simulink model "cv_model_F50"  (R2023a)
settings: Solver=ode23t  StartTime=0  StopTime=6000  FixedStep=0.0005  MaxStep=.01  RelTol=1e-4
model workspace (MAT data in the model file):
  test = 0
values from neighbouring files (symbols this model uses):
  A_cheb_09_1 = [-9.45889157397 1 0 0 0 0 0 0 0 -116.684730988 0 1 ... (81 elements, 9x9)]    [input_reflex_filters.mat]
  B_cheb_09_1 = [1 0 0 0 0 0 0 0 0]    [input_reflex_filters.mat]
  C_cheb_09_1 = [0 0 0 0 0 0 0 0 151338.279895]    [input_reflex_filters.mat]
libraries: SignalEditorBlockLib x4, simulink_extras x4
(part 3 of 4)

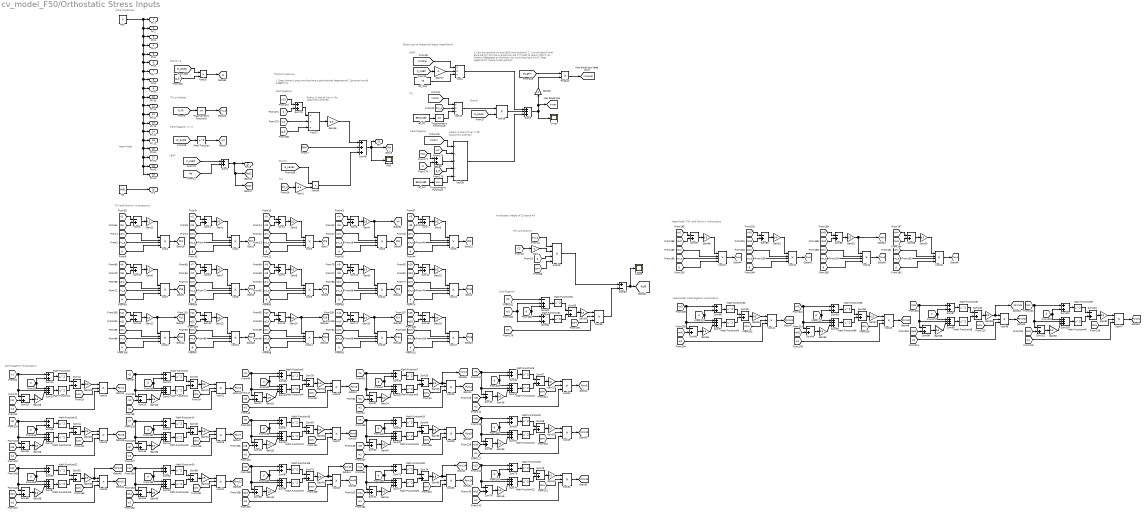
== system cv_model_F50/Orthostatic Stress Inputs ==
  note: Head Model
  note: Centrifugation
  note: Tilt (and Gravity)
  note: Gravity
  note: Tilt
  note: LBNP
  note: Centrifugation
  note: Radius is that of liver (ri for splanchnic arteries).
  note: Gravity
  note: Tilt
  note: Centrifugation: Hydrostatics
  note: 1. Can we combine tilt and LBNP contributions?
      | 2. I've included G level because this formula is empirical, but it stands to reason that if you tilted to 85degrees on the Moon you would lose less fluid
      | 3. Does negative tilt induce hypervolemia?
  note: Hydrostatic Height of CS above AA
  note: Blood Lost to Interstitial Space (Head Down)
  note: Tilt: sin(alpha)
  note: Tilt (and Gravity): Hydrostatics
  note: Initial Conditions
  note: LBNP
  note: Thoracic Pressure
  note: 1. Does thoracic pressure drop have a gravitational dependence? Zamanian would suggest so.
  note: Centrifugation: w^2
  note: Gravity: g
  note: Centrifugation
  note: Radius is that of liver (ri for splanchnic arteries).
  note: Head Model: Tillt (and Gravity) Hydrostatics
  note: Head Model: Centrifugation Hydrostatics
  Gain : Gain  Gain=-1
  Gain1 : Gain  Gain=-3.5  SaturateOnIntegerOverflow=on  OutDataTypeStr=Inherit: Same as input  ParamDataTypeStr=Inherit: Same as input
  Gain{2,5..12,15..16,18..21,23,25..39,41,43..47,49..61} (50 alike) : Gain  Gain=0.5  SaturateOnIntegerOverflow=on  OutDataTypeStr=Inherit: Same as input  ParamDataTypeStr=Inherit: Same as input
  Gain{3..4,13..14,22,24,40,42} (8 alike) : Gain  Gain=1/3  SaturateOnIntegerOverflow=on  OutDataTypeStr=Inherit: Same as input  ParamDataTypeStr=Inherit: Same as input
  Gain17 : Gain  Gain=-1  SaturateOnIntegerOverflow=on  OutDataTypeStr=Inherit: Same as input  ParamDataTypeStr=Inherit: Same as input
  Gain48 : Gain  Gain=-3.5  SaturateOnIntegerOverflow=on  OutDataTypeStr=Inherit: Same as input  ParamDataTypeStr=Inherit: Same as input
  Gain62 : Gain  Gain=-1
  Math Function{,1..40} (41 alike) : Math  Operator=square
  Ph0 : Constant  Value=0
  Product : Product
  Pth1 : Scope
  R0 : Constant  Value=.0001
  Scope : Scope
  Sum{1,4..13,15..19,21,23,25,27,29,31,33,35,37,39,41,43,46,48,50,52,54,56,58,60,62,64,66,68,70,72,74,76,78,83,85..88,90,92,94,96,98,100,102,104} (58 alike) : Sum  Inputs=-+  InputSameDT=on  SaturateOnIntegerOverflow=on  OutDataTypeStr=Inherit: Same as first input
  Sum{2,14,22,26,30,34,38,42,47,51,55,59,63,67,71,75,79..80,84,89,93,97,101} (23 alike) : Sum  InputSameDT=on  SaturateOnIntegerOverflow=on  OutDataTypeStr=Inherit: Same as first input
  Sum{3,20,24,28,32,36,40,44..45,49,53,57,61,65,69,73,77,91,95,99,103} (21 alike) : Sum  Inputs=+++  InputSameDT=on  SaturateOnIntegerOverflow=on  OutDataTypeStr=Inherit: Same as first input
  Sum81 : Sum  Inputs=+-  InputSameDT=on  SaturateOnIntegerOverflow=on  OutDataTypeStr=Inherit: Same as first input
  Sum82 : Sum  Inputs=-++  InputSameDT=on  SaturateOnIntegerOverflow=on  OutDataTypeStr=Inherit: Same as first input
  Trigonometric Function1 : Trigonometry
  Trigonometric Function16 : Trigonometry
  Trigonometric Function2 : Trigonometry
  Vmax : Scope
  kool{1..3,5..14,16..17,19,40..43} (20 alike) : Product  Inputs=****  InputSameDT=on  SaturateOnIntegerOverflow=on  OutDataTypeStr=Inherit: Same as first input
  kool15 : Product  Inputs=**/  InputSameDT=on  SaturateOnIntegerOverflow=on  OutDataTypeStr=Inherit: Same as first input
  kool18 : Product  Inputs=**  InputSameDT=on  SaturateOnIntegerOverflow=on  OutDataTypeStr=Inherit: Same as first input
  kool{20..34,39,44..47} (20 alike) : Product  Inputs=3  InputSameDT=on  SaturateOnIntegerOverflow=on  OutDataTypeStr=Inherit: Same as first input
  kool35 : Product  Inputs=**  InputSameDT=on  SaturateOnIntegerOverflow=on  OutDataTypeStr=Inherit: Same as first input
  kool36 : Product  Inputs=**  InputSameDT=on  SaturateOnIntegerOverflow=on  OutDataTypeStr=Inherit: Same as first input
  kool37 : Product  Inputs=**/  InputSameDT=on  SaturateOnIntegerOverflow=on  OutDataTypeStr=Inherit: Same as first input
  kool38 : Product  Inputs=***//  InputSameDT=on  SaturateOnIntegerOverflow=on  OutDataTypeStr=Inherit: Same as first input
  kool4 : Product  Inputs=**/  InputSameDT=on  SaturateOnIntegerOverflow=on  OutDataTypeStr=Inherit: Same as first input
  ref_lbnp : Constant  Value=70
  ref_src : Constant  Value=85*pi/180
  ref_tilt : Constant  Value=85*pi/180
  Ph.1 : Outport
  Ph.2 : Outport  Port=2
  Ph.3 : Outport  Port=3
  Ph.4 : Outport  Port=4
  Ph.5 : Outport  Port=5
  Ph.6 : Outport  Port=6
  Ph.7 : Outport  Port=7
  Ph.8 : Outport  Port=8
  Ph.9 : Outport  Port=9
  Ph.10 : Outport  Port=10
  Ph.11 : Outport  Port=11
  Ph.12 : Outport  Port=12
  Ph.13 : Outport  Port=13
  Ph.14 : Outport  Port=14
  Ph.15 : Outport  Port=15
  Ph.H1 : Outport  Port=16
  Ph.H2 : Outport  Port=17
  Ph.H3 : Outport  Port=18
  Ph.H4 : Outport  Port=19
  R.0 : Outport  Port=20
  Pth : Outport  Port=21
  Pe.LB : Outport  Port=22
  tag scope: Pe12=global, Pe13=global, Ph10=global, Ph11=global, Ph12=global, Ph13=global, Ph14=global, Ph15=global, Ph1=global, Ph2=global, Ph3=global, Ph4=global, Ph5=global, Ph6=global, Ph7=global, Ph8=global, Ph9=global, PhH1=global, PhH2=global, PhH3=global, PhH4=global, Poff=global, Psrc10=global, Psrc11=global, Psrc12=global, Psrc13=global, Psrc14=global, Psrc15=global, Psrc1=global, Psrc2=global, Psrc3=global, Psrc4=global, Psrc5=global, Psrc6=global, Psrc7=global, Psrc8=global, Psrc9=global, PsrcH1=global, PsrcH2=global, PsrcH3=global, PsrcH4=global, Pth=global, Vmax=global, Vmaxub=global, g=global, h11=global, h13=global, h14=global, h4=global, hH3=global, hsrc11=global, hsrc13=global, hsrc14=global, hsrc4=global, hsrcH3=global, sin_a=global, w2=global
  wires:
  Ph0/1 -> Ph.8/1, Ph.H4/1, Ph.H3/1, Ph.H2/1, Ph.H1/1, Ph.15/1, Ph.14/1, Ph.13/1, Ph.12/1, Ph.11/1, Ph.10/1, Ph.9/1, Ph.7/1, Ph.6/1, Ph.5/1, Ph.4/1, Ph.3/1, Ph.2/1, Ph.1/1
  R0/1 -> R.0/1
  ref_tilt/1 -> Trigonometric Function16/1
  [Vmtilt] -> kool15/1
  Trigonometric Function16/1 -> kool15/3
  [conv] -> kool1/2
  [sin_a] -> kool1/3
  [ri1] -> Sum5/1
  [sin_a] -> kool19/1
  [g] -> kool19/3
  Trigonometric Function2/1 -> [sin_a]
  Gain11/1 -> kool1/1
  Gain/1 -> kool19/2
  [conv] -> kool19/4
  [g] -> kool1/4
  [P_TA] -> Trigonometric Function2/1
  kool1/1 -> [Ph1]
  Sum5/1 -> Gain11/1
  [ro1] -> Sum5/2
  [g] -> kool2/4
  [ri2] -> Sum1/1
  kool2/1 -> [Ph2]
  [conv] -> kool2/2
  [sin_a] -> kool2/3
  Gain2/1 -> kool2/1
  [ro2] -> Sum1/2
  Sum1/1 -> Gain2/1
  Sum4/1 -> Gain3/1
  kool3/1 -> [Ph3]
  [ri3] -> Sum4/1
  [conv] -> kool3/2
  [sin_a] -> kool3/3
  Gain3/1 -> kool3/1
  [ro3] -> Sum4/2
  [g] -> kool3/4
  [g] -> kool5/4
  kool5/1 -> [Ph4]
  Gain4/1 -> [h4], kool5/1
  [ri4] -> Sum6/1
  [sin_a] -> kool5/3
  [ro4] -> Sum6/2
  Sum6/1 -> Gain4/1
  [conv] -> kool5/2
  [sin_a] -> kool6/3
  [ro5] -> Sum7/2
  [ri5] -> Sum7/1
  Gain5/1 -> kool6/1
  [conv] -> kool6/2
  kool6/1 -> [Ph5]
  Sum7/1 -> Gain5/1
  [g] -> kool6/4
  [conv] -> kool10/2
  [ri9] -> Sum11/1
  Gain9/1 -> kool10/1
  kool10/1 -> [Ph9]
  [ri10] -> Sum12/1
  [ro10] -> Sum12/2
  kool11/1 -> [Ph10]
  [g] -> kool10/4
  Sum10/1 -> Gain6/1
  [conv] -> kool11/2
  [ri6] -> Sum10/1
  [g] -> kool9/4
  Gain10/1 -> kool11/1
  [ro8] -> Sum9/2
  Sum11/1 -> Gain9/1
  [conv] -> kool9/2
  [sin_a] -> kool7/3
  kool9/1 -> [Ph8]
  [g] -> kool7/4
  Sum12/1 -> Gain10/1
  Gain8/1 -> kool9/1
  [ri8] -> Sum9/1
  [sin_a] -> kool9/3
  Sum9/1 -> Gain8/1
  kool7/1 -> [Ph6]
  [conv] -> kool7/2
  [sin_a] -> kool10/3
  [ro9] -> Sum11/2
  [g] -> kool11/4
  Gain6/1 -> kool7/1
  [ro6] -> Sum10/2
  Sum8/1 -> Gain7/1
  [sin_a] -> kool11/3
  kool8/1 -> [Ph7]
  [ri7] -> Sum8/1
  [conv] -> kool8/2
  [sin_a] -> kool8/3
  Gain7/1 -> kool8/1
  [ro7] -> Sum8/2
  [g] -> kool8/4
  [conv] -> kool16/2
  [ri14] -> Sum17/1
  Gain15/1 -> [h14], kool16/1
  kool16/1 -> [Ph14]
  [ri15] -> Sum18/1
  [ro15] -> Sum18/2
  kool17/1 -> [Ph15]
  [g] -> kool16/4
  Sum16/1 -> Gain12/1
  [conv] -> kool17/2
  [ri11] -> Sum16/1
  [g] -> kool14/4
  Gain16/1 -> kool17/1
  [ro13] -> Sum15/2
  Sum17/1 -> Gain15/1
  [conv] -> kool14/2
  [sin_a] -> kool12/3
  kool14/1 -> [Ph13]
  [g] -> kool12/4
  Sum18/1 -> Gain16/1
  Gain14/1 -> [h13], kool14/1
  [ri13] -> Sum15/1
  [sin_a] -> kool14/3
  Sum15/1 -> Gain14/1
  kool12/1 -> [Ph11]
  [conv] -> kool12/2
  [sin_a] -> kool16/3
  [ro14] -> Sum17/2
  [g] -> kool17/4
  Gain12/1 -> kool12/1, [h11]
  [ro11] -> Sum16/2
  Sum13/1 -> Gain13/1
  [sin_a] -> kool17/3
  kool13/1 -> [Ph12]
  [ri12] -> Sum13/1
  [conv] -> kool13/2
  [sin_a] -> kool13/3
  Gain13/1 -> kool13/1
  [ro12] -> Sum13/2
  [g] -> kool13/4
  [sin_a] -> Gain1/1
  [sin_a] -> kool15/2
  Sum2/1 -> [Pe13], [Pe12], Pe.LB/1
  [P_LNBP] -> Sum2/1
  [Pe] -> Sum2/2
  [CS] -> Gain/1
  Gain17/1 -> kool4/2
  [Vmlbnp] -> kool4/1
  ref_lbnp/1 -> kool4/3
  Sum3/1 -> Gain62/1, [Vmax], Vmax/1
  kool4/1 -> Sum3/1
  [P_LNBP] -> Gain17/1
  kool15/1 -> kool18/1
  [G_LEVEL] -> kool18/2
  kool18/1 -> Sum3/2
  Math Function/1 -> [w2]
  [W_RADS] -> Math Function/1
  kool20/1 -> [Psrc1]
  [ro1] -> Sum19/2
  Sum19/1 -> Gain18/1
  [ri1] -> Sum14/1, Sum19/1, Sum20/2
  [d] -> Sum20/1, Sum14/2
  Gain18/1 -> Sum20/3
  Sum14/1 -> Math Function1/1
  Sum20/1 -> Math Function2/1
  Math Function2/1 -> Sum21/2
  Math Function1/1 -> Sum21/1
  Sum21/1 -> Gain19/1
  Gain19/1 -> kool20/1
  [conv] -> kool20/2
  [w2] -> kool20/3
  [conv] -> kool21/2
  Sum23/1 -> Gain20/1
  [w2] -> kool21/3
  Sum25/1 -> Gain21/1
  Sum22/1 -> Math Function3/1
  Gain20/1 -> Sum24/3
  Math Function3/1 -> Sum25/1
  Sum24/1 -> Math Function4/1
  kool21/1 -> [Psrc2]
  [ri2] -> Sum22/1, Sum23/1, Sum24/2
  Gain21/1 -> kool21/1
  Math Function4/1 -> Sum25/2
  [ro2] -> Sum23/2
  [d] -> Sum24/1, Sum22/2
  Gain23/1 -> kool22/1
  [ri3] -> Sum26/1, Sum27/1, Sum28/2
  Gain22/1 -> Sum28/3
  Sum28/1 -> Math Function6/1
  Sum26/1 -> Math Function5/1
  Math Function5/1 -> Sum29/1
  Sum29/1 -> Gain23/1
  [d] -> Sum28/1, Sum26/2
  [conv] -> kool22/2
  Sum27/1 -> Gain22/1
  [w2] -> kool22/3
  kool22/1 -> [Psrc3]
  Math Function6/1 -> Sum29/2
  [ro3] -> Sum27/2
  Gain25/1 -> [hsrc4], kool23/1
  [ri4] -> Sum30/1, Sum31/1, Sum32/2
  Gain24/1 -> Sum32/3
  Sum32/1 -> Math Function8/1
  Sum30/1 -> Math Function7/1
  Math Function7/1 -> Sum33/1
  Sum33/1 -> Gain25/1
  [d] -> Sum32/1, Sum30/2
  [conv] -> kool23/2
  Sum31/1 -> Gain24/1
  [w2] -> kool23/3
  kool23/1 -> [Psrc4]
  Math Function8/1 -> Sum33/2
  [ro4] -> Sum31/2
  Gain27/1 -> kool24/1
  [ri5] -> Sum34/1, Sum35/1, Sum36/2
  Gain26/1 -> Sum36/3
  Sum36/1 -> Math Function10/1
  Sum34/1 -> Math Function9/1
  Math Function9/1 -> Sum37/1
  Sum37/1 -> Gain27/1
  [d] -> Sum36/1, Sum34/2
  [conv] -> kool24/2
  Sum35/1 -> Gain26/1
  [w2] -> kool24/3
  kool24/1 -> [Psrc5]
  Math Function10/1 -> Sum37/2
  [ro5] -> Sum35/2
  [ro6] -> Sum39/2
  [conv] -> kool25/2
  Gain28/1 -> Sum40/3
  Sum39/1 -> Gain28/1
  [w2] -> kool25/3
  Sum41/1 -> Gain29/1
  Sum38/1 -> Math Function11/1
  Math Function11/1 -> Sum41/1
  Sum47/1 -> Math Function16/1
  [ri8] -> Sum47/1, Sum48/1, Sum49/2
  Sum49/1 -> Math Function17/1
  Math Function16/1 -> Sum50/1
  Sum50/1 -> Gain33/1
  Gain32/1 -> Sum49/3
  Gain33/1 -> kool27/1
  Math Function13/1 -> Sum41/2
  [conv] -> kool27/2
  [d] -> Sum49/1, Sum47/2
  Math Function17/1 -> Sum50/2
  [ro8] -> Sum48/2
  Sum48/1 -> Gain32/1
  kool29/1 -> [Psrc10]
  Math Function12/1 -> Sum58/2
  [ro10] -> Sum56/2
  [w2] -> kool29/3
  Math Function20/1 -> Sum58/1
  Sum57/1 -> Math Function12/1
  kool27/1 -> [Psrc8]
  Gain36/1 -> Sum57/3
  Sum56/1 -> Gain36/1
  [d] -> Sum57/1, Sum55/2
  kool25/1 -> [Psrc6]
  [d] -> Sum53/1, Sum51/2
  [conv] -> kool29/2
  kool28/1 -> [Psrc9]
  [conv] -> kool28/2
  Sum52/1 -> Gain34/1
  Gain34/1 -> Sum53/3
  Sum54/1 -> Gain35/1
  Sum51/1 -> Math Function18/1
  Gain35/1 -> kool28/1
  Gain37/1 -> kool29/1
  [w2] -> kool28/3
  [ri7] -> Sum42/1, Sum43/1, Sum44/2
  Math Function19/1 -> Sum54/2
  Gain30/1 -> Sum44/3
  Sum55/1 -> Math Function20/1
  Sum44/1 -> Math Function15/1
  Sum42/1 -> Math Function14/1
  Sum53/1 -> Math Function19/1
  Math Function14/1 -> Sum46/1
  Sum46/1 -> Gain31/1
  Math Function18/1 -> Sum54/1
  [w2] -> kool26/3
  kool26/1 -> [Psrc7]
  Sum43/1 -> Gain30/1
  [ri6] -> Sum38/1, Sum39/1, Sum40/2
  Gain31/1 -> kool26/1
  [d] -> Sum44/1, Sum42/2
  Math Function15/1 -> Sum46/2
  Sum58/1 -> Gain37/1
  [ri10] -> Sum55/1, Sum56/1, Sum57/2
  Sum40/1 -> Math Function13/1
  [ro7] -> Sum43/2
  Gain29/1 -> kool25/1
  [ro9] -> Sum52/2
  [d] -> Sum40/1, Sum38/2
  [ri9] -> Sum51/1, Sum52/1, Sum53/2
  [conv] -> kool26/2
  [w2] -> kool27/3
  [ro11] -> Sum60/2
  [conv] -> kool30/2
  Gain38/1 -> Sum61/3
  Sum60/1 -> Gain38/1
  [w2] -> kool30/3
  Sum62/1 -> Gain39/1
  Sum59/1 -> Math Function21/1
  Math Function21/1 -> Sum62/1
  Sum67/1 -> Math Function26/1
  [ri13] -> Sum67/1, Sum68/1, Sum69/2
  Sum69/1 -> Math Function27/1
  Math Function26/1 -> Sum70/1
  Sum70/1 -> Gain43/1
  Gain42/1 -> Sum69/3
  Gain43/1 -> [hsrc13], kool32/1
  Math Function23/1 -> Sum62/2
  [conv] -> kool32/2
  [d] -> Sum69/1, Sum67/2
  Math Function27/1 -> Sum70/2
  [ro13] -> Sum68/2
  Sum68/1 -> Gain42/1
  kool34/1 -> [Psrc15]
  Math Function22/1 -> Sum78/2
  [ro15] -> Sum76/2
  [w2] -> kool34/3
  Math Function30/1 -> Sum78/1
  Sum77/1 -> Math Function22/1
  kool32/1 -> [Psrc13]
  Gain46/1 -> Sum77/3
  Sum76/1 -> Gain46/1
  [d] -> Sum77/1, Sum75/2
  kool30/1 -> [Psrc11]
  [d] -> Sum73/1, Sum71/2
  [conv] -> kool34/2
  kool33/1 -> [Psrc14]
  [conv] -> kool33/2
  Sum72/1 -> Gain44/1
  Gain44/1 -> Sum73/3
  Sum74/1 -> Gain45/1
  Sum71/1 -> Math Function28/1
  Gain45/1 -> [hsrc14], kool33/1
  Gain47/1 -> kool34/1
  [w2] -> kool33/3
  [ri12] -> Sum63/1, Sum64/1, Sum65/2
  Math Function29/1 -> Sum74/2
  Gain40/1 -> Sum65/3
  Sum75/1 -> Math Function30/1
  Sum65/1 -> Math Function25/1
  Sum63/1 -> Math Function24/1
  Sum73/1 -> Math Function29/1
  Math Function24/1 -> Sum66/1
  Sum66/1 -> Gain41/1
  Math Function28/1 -> Sum74/1
  [w2] -> kool31/3
  kool31/1 -> [Psrc12]
  Sum64/1 -> Gain40/1
  [ri11] -> Sum59/1, Sum60/1, Sum61/2
  Gain41/1 -> kool31/1
  [d] -> Sum65/1, Sum63/2
  Math Function25/1 -> Sum66/2
  Sum78/1 -> Gain47/1
  [ri15] -> Sum75/1, Sum76/1, Sum77/2
  Sum61/1 -> Math Function23/1
  [ro12] -> Sum64/2
  Gain39/1 -> [hsrc11], kool30/1
  [ro14] -> Sum72/2
  [d] -> Sum61/1, Sum59/2
  [ri14] -> Sum71/1, Sum72/1, Sum73/2
  [conv] -> kool31/2
  [w2] -> kool32/3
  [G_LEVEL] -> kool35/1
  [g_E] -> kool35/2
  kool35/1 -> [g]
  Gain1/1 -> kool36/2
  [G_LEVEL] -> kool36/1
  [Pth0] -> Sum45/2
  kool36/1 -> Sum45/3
  Sum45/1 -> Pth1/1, [Pth], Pth/1
  [g_E] -> kool37/3
  [w2] -> kool37/2
  Sum79/1 -> kool37/1
  [ri10] -> Sum79/1
  [d] -> Sum79/2
  Gain48/1 -> Sum45/1
  kool37/1 -> Gain48/1
  [w2] -> kool38/2
  [Vmsrc] -> kool38/1
  ref_src/1 -> Trigonometric Function1/1
  Sum80/1 -> kool38/3
  [g_E] -> kool38/4
  Trigonometric Function1/1 -> kool38/5
  [ri10] -> Sum80/1
  [d] -> Sum80/2
  kool38/1 -> Sum3/3
  Sum81/1 -> Scope/1, [Poff]
  kool19/1 -> Sum81/1
  Sum84/1 -> Math Function31/1
  [ro1] -> Sum82/2, Sum84/2
  Sum85/1 -> Gain50/1
  Sum82/1 -> Math Function32/1
  Math Function31/1 -> Sum85/2
  Gain50/1 -> kool39/1
  [d] -> Sum84/1, Sum82/3
  [conv] -> kool39/2
  kool39/1 -> Sum81/2
  [w2] -> kool39/3
  Math Function32/1 -> Sum85/1
  [CS] -> Sum82/1
  kool40/1 -> [PhH1]
  kool43/1 -> [PhH4]
  [conv] -> kool42/2
  [riH2] -> Sum83/1
  Gain53/1 -> kool43/1
  [sin_a] -> kool40/3
  [riH3] -> Sum86/1
  Gain51/1 -> kool41/1
  [roH1] -> Sum87/2
  kool41/1 -> [PhH2]
  [roH3] -> Sum86/2
  Sum83/1 -> Gain51/1
  [riH1] -> Sum87/1
  [roH4] -> Sum88/2
  [conv] -> kool41/2
  [conv] -> kool40/2
  [sin_a] -> kool43/3
  [g] -> kool43/4
  [sin_a] -> kool41/3
  Gain52/1 -> [hH3], kool42/1
  [g] -> kool42/4
  [conv] -> kool43/2
  [sin_a] -> kool42/3
  Gain49/1 -> kool40/1
  [riH4] -> Sum88/1
  kool42/1 -> [PhH3]
  [roH2] -> Sum83/2
  Sum86/1 -> Gain52/1
  [g] -> kool41/4
  [g] -> kool40/4
  Sum87/1 -> Gain49/1
  Sum88/1 -> Gain53/1
  [conv] -> kool47/2
  Sum99/1 -> Math Function38/1
  Sum91/1 -> Math Function34/1
  [w2] -> kool47/3
  Gain60/1 -> Sum103/3
  [w2] -> kool44/3
  Math Function38/1 -> Sum100/2
  [d] -> Sum103/1, Sum101/2
  [conv] -> kool45/2
  Sum92/1 -> Gain55/1
  [w2] -> kool46/3
  Sum98/1 -> Gain58/1
  kool47/1 -> [PsrcH4]
  Sum93/1 -> Math Function35/1
  Math Function39/1 -> Sum104/1
  Sum101/1 -> Math Function39/1
  Gain61/1 -> kool47/1
  Sum95/1 -> Math Function36/1
  Gain56/1 -> Sum95/3
  Sum100/1 -> Gain59/1
  [riH4] -> Sum101/1, Sum102/1, Sum103/2
  [conv] -> kool46/2
  Sum97/1 -> Math Function37/1
  Gain58/1 -> Sum99/3
  [roH4] -> Sum102/2
  Sum102/1 -> Gain60/1
  kool46/1 -> [PsrcH3]
  Sum103/1 -> Math Function40/1
  [d] -> Sum95/1, Sum93/2
  Math Function37/1 -> Sum100/1
  [roH3] -> Sum98/2
  [riH3] -> Sum97/1, Sum98/1, Sum99/2
  Math Function36/1 -> Sum96/2
  Gain57/1 -> kool45/1
  [conv] -> kool44/2
  Gain59/1 -> [hsrcH3], kool46/1
  kool44/1 -> [PsrcH1]
  [roH2] -> Sum94/2
  Sum89/1 -> Math Function33/1
  Gain54/1 -> Sum91/3
  Math Function34/1 -> Sum92/2
  Math Function35/1 -> Sum96/1
  kool45/1 -> [PsrcH2]
  Math Function40/1 -> Sum104/2
  [d] -> Sum91/1, Sum89/2
  [d] -> Sum99/1, Sum97/2
  [riH1] -> Sum89/1, Sum90/1, Sum91/2
  Sum96/1 -> Gain57/1
  Gain55/1 -> kool44/1
  [w2] -> kool45/3
  Sum90/1 -> Gain54/1
  [riH2] -> Sum93/1, Sum94/1, Sum95/2
  Math Function33/1 -> Sum92/1
  Sum104/1 -> Gain61/1
  [roH1] -> Sum90/2
  Sum94/1 -> Gain56/1
  Product/1 -> [Vmaxub]
  Gain62/1 -> Product/2
  [ub_gain] -> Product/1

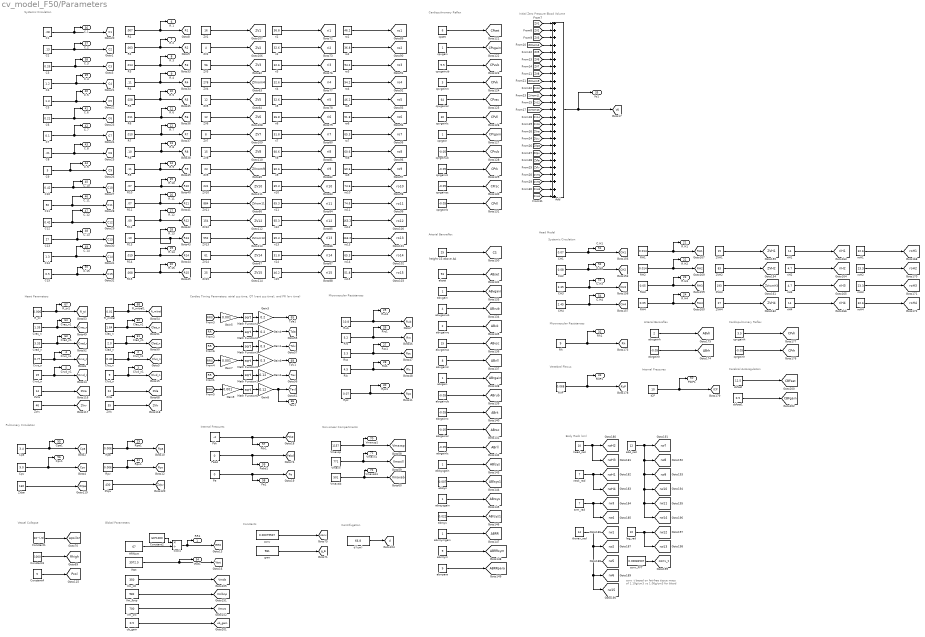
== system cv_model_F50/Parameters ==
  note: Arterial Baroreflex
  note: Systemic Circulation
  note: Microvascular Resistances
  note: Initial Zero Pressure Blood Volume
  note: Cardiopulmonary Reflex
  note: Centrifugation
  note: Constants
  note: Vessel Collapse
  note: Non-Linear Compartments
  note: Heart Parameters
  note: Cardiac Timing Parameters: atrial sys time, QT (vent sys time), and PR (a-v time)
  note: Internal Pressures
  note: Pulmonary Circulation
  note: Microvascular Resistances
  note: Global Parameters
  note: Systemic Circulation
  note: Arterial Baroreflex
  note: Head Model
  note: Cardiopulmonary Reflex
  note: Vertebral Plexus
  note: Internal Pressures
  note: Body Radii (cm)
  note: conv_t based on fat-free tissue mass of 1.10g/cm3 vs 1.06g/cm3 for blood
  note: Cerebral Autoregulation
  Add : Sum  Inputs=+++++++++++++++++++++++++
  C1 : Constant  Value=.28
  C10 : Constant  Value=0.42
  C11 : Constant  Value=50
  C12 : Constant  Value=0.42
  C13 : Constant  Value=27
  C14 : Constant  Value=1.3
  C15 : Constant  Value=0.5
  C2 : Constant  Value=.13
  C3 : Constant  Value=0.26
  C4 : Constant  Value=1.2
  C5 : Constant  Value=1.3
  C6 : Constant  Value=0.21
  C7 : Constant  Value=0.1
  C8 : Constant  Value=.21
  C9 : Constant  Value=5
  CH1 : Constant  Value=0.07
  CH2 : Constant  Value=0.08
  CH3 : Constant  Value=3.35
  CH4 : Constant  Value=2.45
  Clad_n : Constant  Value=2.0
  Clas_n : Constant  Value=1.64
  Clvd_n : Constant  Value=9
  Clvs_n : Constant  Value=0.40
  Constant1 : Constant  Value=10^(-5)
  Constant2 : Constant  Value=60*1000
  Constant3 : Constant  Value=1000
  Constant4 : Constant  Value=5
  Cpa : Constant  Value=3.4
  Cpv : Constant  Value=9.0
  Crad_n : Constant  Value=3.33
  Cras_n : Constant  Value=1.35
  Crvd_n : Constant  Value=19
  Crvs_n : Constant  Value=0.77
  Gain1 : Gain  Gain=0.3
  Gain2 : Gain  Gain=0.12
  Gain3 : Gain  Gain=0.2
  Gain4 : Gain  Gain=0.2
  Gain5 : Gain  Gain=0.001
  Gain6 : Gain  Gain=0.3
  Gain7 : Gain  Gain=0.001
  Gain8 : Gain  Gain=0.12
  Gain9 : Gain  Gain=0.001
  HRNom : Constant  Value=67
  ICP : Constant  Value=10
  Math Function{1..6} (6 alike) : Math  Operator=sqrt  SignedPower=on
  Pabd : Constant  Value=0
  Pe : Constant  Value=0
  Pth : Constant  Value=-4
  R1 : Constant  Value=.007
  R10 : Constant  Value=.07
  R11 : Constant  Value=.07
  R12 : Constant  Value=.09
  R13 : Constant  Value=.10
  R14 : Constant  Value=.019
  R15 : Constant  Value=.008
  R2 : Constant  Value=.003
  R3 : Constant  Value=.014
  R4 : Constant  Value=.11
  R5 : Constant  Value=.028
  R6 : Constant  Value=.011
  R7 : Constant  Value=.010
  R8 : Constant  Value=.10
  R9 : Constant  Value=.11
  RH1 : Constant  Value=0.014
  RH2 : Constant  Value=0.014
  RH3 : Constant  Value=0.05
  RH4 : Constant  Value=0.05
  RVP : Constant  Value=0.068
  R_mitral : Constant  Value=0.01
  R_tri : Constant  Value=0.006
  Rh : Constant  Value=9
  Rlc : Constant  Value=4.5
  Rpa : Constant  Value=0.006
  Rpc : Constant  Value=0.07
  Rpv : Constant  Value=0.006
  Rrc : Constant  Value=5.2
  Rsc : Constant  Value=3.3
  Rub : Constant  Value=10.8
  Vm_lbnp : Constant  Value=982
  Vm_src : Constant  Value=700
  Vm_tilt : Constant  Value=350
  Vmaxab : Constant  Value=501
  Vmaxll : Constant  Value=771
  Vmaxsp : Constant  Value=1157
  Vtot : Constant  Value=3972.5
  ZV1 : Constant  Value=16
  ZV10 : Constant  Value=231
  ZV11 : Constant  Value=884
  ZV12 : Constant  Value=154
  ZV13 : Constant  Value=552
  ZV14 : Constant  Value=61
  ZV15 : Constant  Value=25
  ZV2 : Constant  Value=4
  ZV3 : Constant  Value=56
  ZV4 : Constant  Value=278
  ZV5 : Constant  Value=12
  ZV6 : Constant  Value=12
  ZV7 : Constant  Value=8
  ZV8 : Constant  Value=15
  ZV9 : Constant  Value=23
  ZVH1 : Constant  Value=15
  ZVH2 : Constant  Value=83
  ZVH3 : Constant  Value=193
  ZVH4 : Constant  Value=27
  ZVla : Constant  Value=24
  ZVlv : Constant  Value=55
  ZVpa : Constant  Value=160
  ZVpv : Constant  Value=430
  ZVra : Constant  Value=14
  ZVrv : Constant  Value=46
  abd_rad : Constant  Value=12
  ablsys : Constant  Value=0.007
  ablsysgain : Constant
  abrgain : Constant
  abrgainh : Constant  Value=-0.05
  abrgainlc : Constant  Value=-0.05
  abrgainrc : Constant  Value=-0.05
  abrgainsc : Constant  Value=-0.05
  abrgainub : Constant  Value=-0.05
  abrrpara : Constant  Value=9
  abrrsym : Constant  Value=9
  abrrsymgain : Constant
  abrsys : Constant  Value=0.022
  abrsysgain : Constant
  abset : Constant  Value=93
  abvgain : Constant
  abvgainh : Constant  Value=2
  abvgainlc : Constant  Value=8
  abvgainrc : Constant  Value=2
  abvgainsc : Constant  Value=15
  abvgainub : Constant  Value=4
  arm_rad : Constant  Value=7
  cbfset : Constant  Value=12.5
  cbfset1 : Constant  Value=0.5
  conv : Constant  Value=0.00079507
  conv_FFT : Constant  Value=0.00082507
  cprgain : Constant
  cprgainh : Constant  Value=-0.05
  cprgainlc : Constant  Value=-0.05
  cprgainrc : Constant  Value=-0.05
  cprgainsc : Constant  Value=-0.05
  cprgainub : Constant  Value=-0.05
  cpset : Constant  Value=6
  cpvgain : Constant
  cpvgainh : Constant  Value=3.5
  cpvgainlc : Constant  Value=30
  cpvgainrc : Constant  Value=3
  cpvgainsc : Constant  Value=64
  cpvgainub : Constant  Value=9.5
  d (cm) : Constant  Value=66.8
  grav : Constant  Value=981
  head_rad : Constant  Value=10
  height CS above AA : Constant  Value=25
  kool1 : Product  Inputs=*/  InputSameDT=on  SaturateOnIntegerOverflow=on  OutDataTypeStr=Inherit: Same as first input
  leg_rad : Constant  Value=10
  neck_rad : Constant  Value=7
  ri1 : Constant  Value=36.8
  ri{10..13} (4 alike) : Constant  Value=65.3
  ri14 : Constant  Value=51.8
  ri15 : Constant  Value=46.2
  ri{2..5} (4 alike) : Constant  Value=32.6
  ri6 : Constant  Value=36.8
  ri7 : Constant  Value=51.8
  ri8 : Constant  Value=60.6
  ri9 : Constant  Value=60.6
  riH1 : Constant  Value=14
  riH2 : Constant  Value=4.7
  riH3 : Constant  Value=4.7
  riH4 : Constant  Value=14
  ro1 : Constant  Value=46.2
  ro10 : Constant  Value=74.6
  ro11 : Constant  Value=74.6
  ro12 : Constant  Value=163.2
  ro13 : Constant  Value=163.2
  ro14 : Constant  Value=65.3
  ro15 : Constant  Value=51.8
  ro2 : Constant  Value=36.8
  ro3 : Constant  Value=94.2
  ro4 : Constant  Value=94.2
  ro5 : Constant  Value=46.2
  ro6 : Constant  Value=51.8
  ro7 : Constant  Value=65.3
  ro8 : Constant  Value=60.6
  ro9 : Constant  Value=60.6
  roH1 : Constant  Value=32.6
  roH2 : Constant  Value=23.3
  roH3 : Constant  Value=23.3
  roH4 : Constant  Value=32.6
  thorax_rad : Constant  Value=14
  ub_gain : Constant  Value=0.5
  RR1 : Outport
  Clvs_n1 : Outport  Port=2
  Clvd_n1 : Outport  Port=3
  Crvs_n1 : Outport  Port=4
  Crvd_n1 : Outport  Port=5
  R.1 : Outport  Port=6
  R.2 : Outport  Port=7
  R.3 : Outport  Port=8
  R.4 : Outport  Port=9
  R.5 : Outport  Port=10
  R.6 : Outport  Port=11
  R.7 : Outport  Port=12
  R.8 : Outport  Port=13
  R.9 : Outport  Port=14
  R.10 : Outport  Port=15
  R.11 : Outport  Port=16
  R.12 : Outport  Port=17
  R.13 : Outport  Port=18
  R.14 : Outport  Port=19
  R.15 : Outport  Port=20
  R.H1 : Outport  Port=21
  R.H2 : Outport  Port=22
  R.H3 : Outport  Port=23
  R.H4 : Outport  Port=24
  Rub1 : Outport  Port=25
  Rrc1 : Outport  Port=26
  Rsc1 : Outport  Port=27
  Rlc1 : Outport  Port=28
  Rpa1 : Outport  Port=29
  Rpc1 : Outport  Port=30
  Rpv1 : Outport  Port=31
  Rh1 : Outport  Port=32
  RVP1 : Outport  Port=33
  Vtot1 : Outport  Port=34
  Vo1 : Outport  Port=35
  C.1 : Outport  Port=36
  C.2 : Outport  Port=37
  C.3 : Outport  Port=38
  C.4 : Outport  Port=39
  C.5 : Outport  Port=40
  C.6 : Outport  Port=41
  C.7 : Outport  Port=42
  C.8 : Outport  Port=43
  C.9 : Outport  Port=44
  C.10 : Outport  Port=45
  C.11 : Outport  Port=46
  C.12 : Outport  Port=47
  C.13 : Outport  Port=48
  C.14 : Outport  Port=49
  C.15 : Outport  Port=50
  C.H1 : Outport  Port=51
  C.H2 : Outport  Port=52
  C.H3 : Outport  Port=53
  C.H4 : Outport  Port=54
  Cpa1 : Outport  Port=55
  Cpv1 : Outport  Port=56
  Pth1 : Outport  Port=57
  Pe1 : Outport  Port=58
  Pabd1 : Outport  Port=59
  PICP1 : Outport  Port=60
  Clad_n1 : Outport  Port=61
  Clas_n1 : Outport  Port=62
  Crad_n1 : Outport  Port=63
  Cras_n1 : Outport  Port=64
  Tsla1 : Outport  Port=65
  Tav1 : Outport  Port=66
  R_tri1 : Outport  Port=67
  R_mitral1 : Outport  Port=68
  Tslv1 : Outport  Port=69
  Vmaxsp1 : Outport  Port=70
  Vmaxll1 : Outport  Port=71
  Vmaxab1 : Outport  Port=72
  tag scope: ABRR=global, ABRRpara=global, ABRRsym=global, ABlsys1=global, ABlsys=global, ABrgain=global, ABrh=global, ABrk=global, ABrll=global, ABrsc=global, ABrsys1=global, ABrsys=global, ABrub=global, ABset=global, ABvgain=global, ABvh=global, ABvk=global, ABvll=global, ABvsc=global, ABvub=global, C10=global, C11=global, C12=global, C13=global, C14=global, C15=global, C1=global, C2=global, C3=global, C4=global, C5=global, C6=global, C7=global, C8=global, C9=global, CBFgain=global, CBFset=global, CH1=global, CH2=global, CH3=global, CH4=global, CPrgain=global, CPrh=global, CPrk=global, CPrll=global, CPrsc=global, CPrub=global, CPset=global, CPvgain=global, CPvh=global, CPvk=global, CPvll=global, CPvsc=global, CPvub=global, CS=global, Clad_n=global, Clas_n=global, Clvd_n=global, Clvs_n=global, Cpa=global, Cpv=global, Crad_n=global, Cras_n=global, Crvd_n=global, Crvs_n=global, ICP=global, Pabd=global, Pcol=global, Pe=global, Pth0=global, R10=global, R11=global, R12=global, R13=global, R14=global, R15=global, R1=global, R2=global, R3=global, R4=global, R5=global, R6=global, R7=global, R8=global, R9=global, RH1=global, RH2=global, RH3=global, RH4=global, RR0=global, RVP=global, R_mitral=global, R_tri=global, Rh=global, Rhigh=global, Rlc=global, Rpa=global, Rpc=global, Rpv=global, Rrc=global, Rsc=global, Rub=global, Tav0=global, Tav=global, Tsla=global, Tslv=global, V0=global, Vmaxab=global, Vmaxll=global, Vmaxsp=global, Vmlbnp=global, Vmsrc=global, Vmtilt=global, Vtot=global, ZV10=global, ZV12=global, ZV14=global, ZV15=global, ZV1=global, ZV2=global, ZV3=global, ZV5=global, ZV6=global, ZV7=global, ZV8=global, ZVH1=global, ZVH2=global, ZVH4=global, ZVla=global, ZVlv=global, ZVnom11=global, ZVnom13=global, ZVnom4=global, ZVnom9=global, ZVnomH3=global, ZVpa=global, ZVpv=global, ZVra=global, ZVrv=global, conv=global, conv_t=global, d=global, epsilon=global, g_E=global, ri10=global, ri11=global, ri12=global, ri13=global, ri14=global, ri15=global, ri1=global, ri2=global, ri3=global, ri4=global, ri5=global, ri6=global, ri7=global, ri8=global, ri9=global, riH1=global, riH2=global, riH3=global, riH4=global, ro10=global, ro11=global, ro12=global, ro13=global, ro14=global, ro15=global, ro1=global, ro2=global, ro3=global, ro4=global, ro5=global, ro6=global, ro7=global, ro8=global, ro9=global, roH1=global, roH2=global, roH3=global, roH4=global, rw10=global, rw11=global, rw12=global, rw13=global, rw14=global, rw15=global, rw1=global, rw2=global, rw3=global, rw4=global, rw5=global, rw6=global, rw7=global, rw8=global, rw9=global, rwH1=global, rwH2=global, rwH3=global, rwH4=global, ub_gain=global
  wires:
  Cpa/1 -> [Cpa], Cpa1/1
  Cpv/1 -> [Cpv], Cpv1/1
  Clvs_n/1 -> Clvs_n1/1, [Clvs_n]
  Crvs_n/1 -> [Crvs_n], Crvs_n1/1
  Rpa/1 -> Rpa1/1, [Rpa]
  Rpc/1 -> [Rpc], Rpc1/1
  Rpv/1 -> Rpv1/1, [Rpv]
  Crvd_n/1 -> [Crvd_n], Crvd_n1/1
  Clvd_n/1 -> Clvd_n1/1, [Clvd_n]
  Add/1 -> Vo1/1, [V0]
  Pth/1 -> Pth1/1, [Pth0]
  C1/1 -> [C1], C.1/1
  C2/1 -> [C2], C.2/1
  C3/1 -> [C3], C.3/1
  C4/1 -> [C4], C.4/1
  C5/1 -> C.5/1, [C5]
  C6/1 -> C.6/1, [C6]
  C7/1 -> C.7/1, [C7]
  C8/1 -> [C8], C.8/1
  C9/1 -> C.9/1, [C9]
  C10/1 -> C.10/1, [C10]
  C11/1 -> C.11/1, [C11]
  C12/1 -> C.12/1, [C12]
  C13/1 -> [C13], C.13/1
  C14/1 -> [C14], C.14/1
  R1/1 -> [R1], R.1/1
  R2/1 -> [R2], R.2/1
  R3/1 -> [R3], R.3/1
  R4/1 -> [R4], R.4/1
  R5/1 -> [R5], R.5/1
  R6/1 -> [R6], R.6/1
  R7/1 -> [R7], R.7/1
  R8/1 -> [R8], R.8/1
  R9/1 -> [R9], R.9/1
  R10/1 -> [R10], R.10/1
  R11/1 -> [R11], R.11/1
  R12/1 -> [R12], R.12/1
  R13/1 -> R.13/1, [R13]
  R14/1 -> [R14], R.14/1
  R15/1 -> [R15], R.15/1
  Rub/1 -> Rub1/1, [Rub]
  Rrc/1 -> [Rrc], Rrc1/1
  Rsc/1 -> [Rsc], Rsc1/1
  Rlc/1 -> [Rlc], Rlc1/1
  C15/1 -> C.15/1, [C15]
  Pe/1 -> Pe1/1, [Pe]
  Cras_n/1 -> [Cras_n], Cras_n1/1
  Clad_n/1 -> [Clad_n], Clad_n1/1
  Crad_n/1 -> Crad_n1/1, [Crad_n]
  R_tri/1 -> [R_tri], R_tri1/1
  R_mitral/1 -> [R_mitral], R_mitral1/1
  Math Function3/1 -> Gain1/1
  [RR] -> Math Function3/1
  Gain1/1 -> [Tslv]
  Gain2/1 -> [Tav]
  Math Function2/1 -> Gain4/1
  [RR] -> Math Function2/1
  Gain4/1 -> [Tsla]
  Math Function1/1 -> Gain2/1
  [RR] -> Math Function1/1
  Clas_n/1 -> [Clas_n], Clas_n1/1
  Vmaxsp/1 -> [Vmaxsp], Vmaxsp1/1
  Vmaxll/1 -> Vmaxll1/1, [Vmaxll]
  Vmaxab/1 -> Vmaxab1/1, [Vmaxab]
  Math Function4/1 -> Gain3/1
  [RR0] -> Gain5/1
  Gain5/1 -> Math Function4/1
  Gain3/1 -> Tsla1/1
  Math Function5/1 -> Gain6/1
  [RR0] -> Gain7/1
  Gain7/1 -> Math Function5/1
  Gain6/1 -> Tslv1/1
  Math Function6/1 -> Gain8/1
  [RR0] -> Gain9/1
  Gain9/1 -> Math Function6/1
  Gain8/1 -> Tav1/1, [Tav0]
  ZV3/1 -> [ZV3]
  ZV4/1 -> [ZVnom4]
  ZV5/1 -> [ZV5]
  ZV9/1 -> [ZVnom9]
  ZV11/1 -> [ZVnom11]
  ZV14/1 -> [ZV14]
  ZVla/1 -> [ZVla]
  Constant3/1 -> [Rhigh]
  Constant1/1 -> [epsilon]
  Vtot/1 -> [Vtot], Vtot1/1
  Pabd/1 -> [Pabd], Pabd1/1
  conv/1 -> [conv]
  Constant2/1 -> kool1/1
  HRNom/1 -> kool1/2
  kool1/1 -> [RR0], RR1/1
  ri1/1 -> [ri1]
  ri2/1 -> [ri2]
  ri3/1 -> [ri3]
  ri4/1 -> [ri4]
  ri5/1 -> [ri5]
  ri6/1 -> [ri6]
  ri7/1 -> [ri7]
  ri8/1 -> [ri8]
  ri9/1 -> [ri9]
  ri10/1 -> [ri10]
  ri11/1 -> [ri11]
  ri12/1 -> [ri12]
  ri13/1 -> [ri13]
  ri14/1 -> [ri14]
  ri15/1 -> [ri15]
  ro1/1 -> [ro1]
  ro2/1 -> [ro2]
  ro3/1 -> [ro3]
  ro4/1 -> [ro4]
  ro5/1 -> [ro5]
  ro6/1 -> [ro6]
  ro7/1 -> [ro7]
  ro8/1 -> [ro8]
  ro9/1 -> [ro9]
  ro10/1 -> [ro10]
  ro11/1 -> [ro11]
  ro12/1 -> [ro12]
  ro13/1 -> [ro13]
  ro14/1 -> [ro14]
  ro15/1 -> [ro15]
  d (cm)/1 -> [d]
  Vm_tilt/1 -> [Vmtilt]
  grav/1 -> [g_E]
  ZV2/1 -> [ZV2]
  ZV1/1 -> [ZV1]
  ZV6/1 -> [ZV6]
  ZV7/1 -> [ZV7]
  ZV8/1 -> [ZV8]
  ZV10/1 -> [ZV10]
  ZV12/1 -> [ZV12]
  ZV13/1 -> [ZVnom13]
  ZV15/1 -> [ZV15]
  Constant4/1 -> [Pcol]
  ZVra/1 -> [ZVra]
  ZVrv/1 -> [ZVrv]
  ZVlv/1 -> [ZVlv]
  ZVpa/1 -> [ZVpa]
  ZVpv/1 -> [ZVpv]
  cpset/1 -> [CPset]
  cpvgain/1 -> [CPvgain]
  cpvgainub/1 -> [CPvub]
  cpvgainrc/1 -> [CPvk]
  cpvgainsc/1 -> [CPvsc]
  cpvgainlc/1 -> [CPvll]
  cprgain/1 -> [CPrgain]
  cprgainub/1 -> [CPrub]
  cprgainrc/1 -> [CPrk]
  cprgainsc/1 -> [CPrsc]
  cprgainlc/1 -> [CPrll]
  abrgainub/1 -> [ABrub]
  abrgainrc/1 -> [ABrk]
  abvgainlc/1 -> [ABvll]
  abset/1 -> [ABset]
  abvgainrc/1 -> [ABvk]
  abvgainub/1 -> [ABvub]
  abvgainsc/1 -> [ABvsc]
  abvgain/1 -> [ABvgain]
  abrgain/1 -> [ABrgain]
  abrgainlc/1 -> [ABrll]
  abrgainsc/1 -> [ABrsc]
  ablsysgain/1 -> [ABlsys]
  ablsys/1 -> [ABlsys1]
  abrsysgain/1 -> [ABrsys]
  abrsys/1 -> [ABrsys1]
  abrrpara/1 -> [ABRRpara]
  abrrsym/1 -> [ABRRsym]
  abrrsymgain/1 -> [ABRR]
  height CS above AA/1 -> [CS]
  [ZV1] -> Add/1
  [ZV2] -> Add/2
  [ZV3] -> Add/3
  [ZVnom4] -> Add/4
  [ZV5] -> Add/5
  [ZV6] -> Add/6
  [ZV7] -> Add/7
  [ZV8] -> Add/8
  [ZVnom9] -> Add/9
  [ZV10] -> Add/10
  [ZVnom11] -> Add/11
  [ZV12] -> Add/12
  [ZVnom13] -> Add/13
  [ZV14] -> Add/14
  [ZV15] -> Add/15
  [ZVra] -> Add/16
  [ZVrv] -> Add/17
  [ZVpa] -> Add/18
  [ZVpv] -> Add/19
  [ZVla] -> Add/20
  [ZVlv] -> Add/21
  Vm_lbnp/1 -> [Vmlbnp]
  Vm_src/1 -> [Vmsrc]
  ZVH4/1 -> [ZVH4]
  roH3/1 -> [roH3]
  RH4/1 -> [RH4], R.H4/1
  roH1/1 -> [roH1]
  roH4/1 -> [roH4]
  RH2/1 -> [RH2], R.H2/1
  ZVH1/1 -> [ZVH1]
  ZVH2/1 -> [ZVH2]
  riH1/1 -> [riH1]
  roH2/1 -> [roH2]
  riH4/1 -> [riH4]
  riH3/1 -> [riH3]
  RH1/1 -> [RH1], R.H1/1
  RH3/1 -> [RH3], R.H3/1
  CH4/1 -> [CH4], C.H4/1
  CH1/1 -> [CH1], C.H1/1
  ZVH3/1 -> [ZVnomH3]
  CH2/1 -> [CH2], C.H2/1
  CH3/1 -> [CH3], C.H3/1
  riH2/1 -> [riH2]
  [ZVH1] -> Add/22
  [ZVH4] -> Add/25
  [ZVH3] -> Add/24
  [ZVH2] -> Add/23
  Rh/1 -> Rh1/1, [Rh]
  abrgainh/1 -> [ABrh]
  abvgainh/1 -> [ABvh]
  cpvgainh/1 -> [CPvh]
  cprgainh/1 -> [CPrh]
  RVP/1 -> RVP1/1, [RVP]
  ICP/1 -> PICP1/1, [ICP]
  head_rad/1 -> [rwH3], [rwH2]
  neck_rad/1 -> [rwH4], [rwH1]
  arm_rad/1 -> [rw4], [rw3]
  thorax_rad/1 -> [rw15], [rw6], [rw5], [rw2], [rw1]
  abd_rad/1 -> [rw14], [rw11], [rw10], [rw9], [rw8], [rw7]
  leg_rad/1 -> [rw13], [rw12]
  conv_FFT/1 -> [conv_t]
  cbfset/1 -> [CBFset]
  ub_gain/1 -> [ub_gain]
  cbfset1/1 -> [CBFgain]

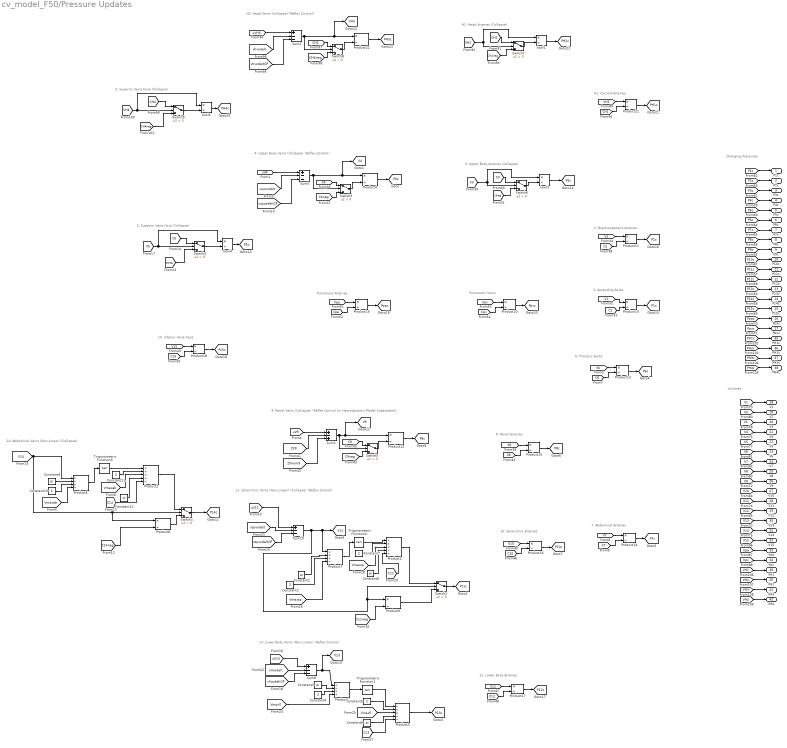
== system cv_model_F50/Pressure Updates ==
  note: 11: Splanchnic Veins (Non-Linear) (Collapse) (Reflex Control)
  note: 14: Abdominal Veins (Non-Linear) (Collapse)
  note: 13: Lower Body Veins (Non-Linear) (Reflex Control)
  note: 10: Splanchnic Arteries
  note: 15: Inferior Vena Cava
  note: 12: Lower Body Arteries
  note: Pulmonary Arteries
  note: Pulmonary Veins
  note: 9: Renal Veins (Collapse) (Reflex Control [in Hemodynamic Model Subsystem])
  note: 8: Renal Arteries
  note: 7: Abdominal Arteries
  note: 6: Thoracic Aorta
  note: 5: Superior Vena Cava (Collapse)
  note: 4: Upper Body Veins (Collapse) (Reflex Control)
  note: 3: Upper Body Arteries (Collapse)
  note: 2: Brachiocephalic Arteries
  note: 1: Ascending Aorta
  note: Volumes
  note: Changing Pressures
  note: H1: Carotid Arteries
  note: H2: Head Arteries (Collapse)
  note: H3: Head Veins (Collapse) (Reflex Control)
  note: 5: Superior Vena Cava (Collapse)
  Constant{1,3,6,8..9,12} (6 alike) : Constant  Value=pi
  Constant{2,4..5,7,10..11} (6 alike) : Constant  Value=2
  Product1 : Product  Inputs=***//  SaturateOnIntegerOverflow=on  OutDataTypeStr=Inherit: Same as first input
  Product{4,8..22} (16 alike) : Product  Inputs=*/  SaturateOnIntegerOverflow=on  OutDataTypeStr=Inherit: Same as first input
  Product2 : Product  Inputs=***//  SaturateOnIntegerOverflow=on  OutDataTypeStr=Inherit: Same as first input
  Product3 : Product  Inputs=***//  SaturateOnIntegerOverflow=on  OutDataTypeStr=Inherit: Same as first input
  Product5 : Product  Inputs=**//  SaturateOnIntegerOverflow=on  OutDataTypeStr=Inherit: Same as first input
  Product6 : Product  Inputs=**//  SaturateOnIntegerOverflow=on  OutDataTypeStr=Inherit: Same as first input
  Product7 : Product  Inputs=**//  SaturateOnIntegerOverflow=on  OutDataTypeStr=Inherit: Same as first input
  Sum1 : Sum  Inputs=+-+  InputSameDT=on  SaturateOnIntegerOverflow=on  OutDataTypeStr=Inherit: Same as first input
  Sum{2,5,8,10} (4 alike) : Sum  Inputs=+--  InputSameDT=on  SaturateOnIntegerOverflow=on  OutDataTypeStr=Inherit: Same as first input
  Switch{1..9} (9 alike) : Switch  Criteria=u2 > Threshold
  Trigonometric Function1 : Trigonometry  Operator=tan
  Trigonometric Function2 : Trigonometry  Operator=tan
  Trigonometric Function3 : Trigonometry  Operator=tan
  kool{1..4} (4 alike) : Product  Inputs=*/  InputSameDT=on  SaturateOnIntegerOverflow=on  OutDataTypeStr=Inherit: Same as first input
  P1c : Outport
  P2c : Outport  Port=2
  P3c : Outport  Port=3
  P4c : Outport  Port=4
  P5c : Outport  Port=5
  P6c : Outport  Port=6
  P7c : Outport  Port=7
  P8c : Outport  Port=8
  P9c : Outport  Port=9
  P10c : Outport  Port=10
  P11c : Outport  Port=11
  P12c : Outport  Port=12
  P13c : Outport  Port=13
  P14c : Outport  Port=14
  P15c : Outport  Port=15
  Ppac : Outport  Port=16
  Ppvc : Outport  Port=17
  V1 : Outport  Port=18
  V2 : Outport  Port=19
  V3 : Outport  Port=20
  V4 : Outport  Port=21
  V5 : Outport  Port=22
  V6 : Outport  Port=23
  V7 : Outport  Port=24
  V8 : Outport  Port=25
  V9 : Outport  Port=26
  V10 : Outport  Port=27
  V11 : Outport  Port=28
  V12 : Outport  Port=29
  V13 : Outport  Port=30
  V14 : Outport  Port=31
  V15 : Outport  Port=32
  Vpa : Outport  Port=33
  Vpv : Outport  Port=34
  PH1c : Outport  Port=35
  PH2c : Outport  Port=36
  PH3c : Outport  Port=37
  PH4c : Outport  Port=38
  VH1 : Outport  Port=39
  VH2 : Outport  Port=40
  VH3 : Outport  Port=41
  VH4 : Outport  Port=42
  tag scope: P10c=global, P11c=global, P12c=global, P13c=global, P14c=global, P15c=global, P1c=global, P2c=global, P3c=global, P4c=global, P5c=global, P6c=global, P7c=global, P8c=global, P9c=global, PH1c=global, PH2c=global, PH3c=global, PH4c=global, Ppac=global, Ppvc=global, V11=global, V13=global, V4=global, V9=global, VH3=global
  wires:
  Product3/1 -> [P13c]
  [vllvodelt] -> Sum8/2
  [vllvodeltCP] -> Sum8/3
  Sum8/1 -> [V13], Product6/1
  [uV13] -> Sum8/1
  Constant3/1 -> Product6/2
  Constant4/1 -> Product6/3
  [Vmaxll] -> Product6/4
  Product6/1 -> Trigonometric Function1/1
  Trigonometric Function1/1 -> Product3/1
  Constant5/1 -> Product3/2
  [Vmaxll] -> Product3/3
  Constant6/1 -> Product3/4
  [C13] -> Product3/5
  [vspvodelt] -> Sum10/2
  [vspvodeltCP] -> Sum10/3
  Sum10/1 -> Product9/1, Switch2/2, Product7/1, [V11]
  [uV11] -> Sum10/1
  [vupvodeltCP] -> Sum5/3
  [uV4] -> Sum5/1
  Sum5/1 -> Switch3/2, Product4/1, [V4]
  Product4/1 -> [P4c]
  [ZV9] -> Sum1/2
  [ZVnom9] -> Sum1/3
  [uV9] -> Sum1/1
  Sum1/1 -> Switch5/2, Product12/1, [V9]
  Product12/1 -> [P9c]
  [C9] -> Switch5/1
  [C9neg] -> Switch5/3
  Switch5/1 -> Product12/2
  [C4] -> Switch3/1
  [C4neg] -> Switch3/3
  Switch3/1 -> Product4/2
  Product1/1 -> Switch2/1
  Constant1/1 -> Product7/2
  Constant2/1 -> Product7/3
  [Vmaxsp] -> Product7/4
  Product7/1 -> Trigonometric Function2/1
  Trigonometric Function2/1 -> Product1/1
  Constant7/1 -> Product1/2
  [Vmaxsp] -> Product1/3
  Constant8/1 -> Product1/4
  [C11] -> Product1/5
  Switch2/1 -> [P11c]
  [C11neg] -> Product9/2
  Product9/1 -> Switch2/3
  [V14] -> Product8/1, Switch1/2, Product5/1
  Product2/1 -> Switch1/1
  Constant9/1 -> Product5/2
  Constant10/1 -> Product5/3
  [Vmaxab] -> Product5/4
  Product5/1 -> Trigonometric Function3/1
  Trigonometric Function3/1 -> Product2/1
  Constant11/1 -> Product2/2
  [Vmaxab] -> Product2/3
  Constant12/1 -> Product2/4
  [C14] -> Product2/5
  Switch1/1 -> [P14c]
  [C14neg] -> Product8/2
  Product8/1 -> Switch1/3
  [V5] -> Switch4/2, kool4/1
  [C5] -> Switch4/1
  [C5neg] -> Switch4/3
  Switch4/1 -> kool4/2
  kool4/1 -> [P5c]
  [V3] -> Switch6/2, kool3/1
  [C3] -> Switch6/1
  [C3neg] -> Switch6/3
  Switch6/1 -> kool3/2
  kool3/1 -> [P3c]
  [V1] -> Product10/1
  [C1] -> Product10/2
  Product10/1 -> [P1c]
  [V2] -> Product11/1
  [C2] -> Product11/2
  Product11/1 -> [P2c]
  [V6] -> Product13/1
  [C6] -> Product13/2
  Product13/1 -> [P6c]
  [V7] -> Product14/1
  [C7] -> Product14/2
  Product14/1 -> [P7c]
  [V8] -> Product15/1
  [C8] -> Product15/2
  Product15/1 -> [P8c]
  [V10] -> Product16/1
  [C10] -> Product16/2
  Product16/1 -> [P10c]
  [V12] -> Product17/1
  [C12] -> Product17/2
  Product17/1 -> [P12c]
  [V15] -> Product18/1
  [C15] -> Product18/2
  Product18/1 -> [P15c]
  [Vpa] -> Product19/1
  [Cpa] -> Product19/2
  Product19/1 -> [Ppac]
  [Vpv] -> Product20/1
  [Cpv] -> Product20/2
  Product20/1 -> [Ppvc]
  [P1c] -> P1c/1
  [P2c] -> P2c/1
  [P3c] -> P3c/1
  [P4c] -> P4c/1
  [P5c] -> P5c/1
  [P6c] -> P6c/1
  [P7c] -> P7c/1
  [P8c] -> P8c/1
  [P9c] -> P9c/1
  [P10c] -> P10c/1
  [P11c] -> P11c/1
  [P12c] -> P12c/1
  [P13c] -> P13c/1
  [P14c] -> P14c/1
  [P15c] -> P15c/1
  [Ppac] -> Ppac/1
  [Ppvc] -> Ppvc/1
  [Vpv] -> Vpv/1
  [Vpa] -> Vpa/1
  [V4] -> V4/1
  [V15] -> V15/1
  [V12] -> V12/1
  [V13] -> V13/1
  [V14] -> V14/1
  [V2] -> V2/1
  [V1] -> V1/1
  [V10] -> V10/1
  [V11] -> V11/1
  [V9] -> V9/1
  [V7] -> V7/1
  [V6] -> V6/1
  [V5] -> V5/1
  [V8] -> V8/1
  [V3] -> V3/1
  [vupvodelt] -> Sum5/2
  [CH1] -> Product21/2
  [VH1] -> Product21/1
  Product21/1 -> [PH1c]
  Switch7/1 -> kool1/2
  [VH2] -> Switch7/2, kool1/1
  kool1/1 -> [PH2c]
  [CH2neg] -> Switch7/3
  [CH2] -> Switch7/1
  [vhvodeltCP] -> Sum2/3
  Product22/1 -> [PH3c]
  Switch8/1 -> Product22/2
  [CH4] -> Switch8/1
  Sum2/1 -> Switch8/2, Product22/1, [VH3]
  [CH4neg] -> Switch8/3
  [uVH3] -> Sum2/1
  [vhvodelt] -> Sum2/2
  [CH4] -> Switch9/1
  [VH4] -> Switch9/2, kool2/1
  Switch9/1 -> kool2/2
  [CH4neg] -> Switch9/3
  kool2/1 -> [PH4c]
  [PH4c] -> PH4c/1
  [PH2c] -> PH2c/1
  [PH3c] -> PH3c/1
  [PH1c] -> PH1c/1
  [VH2] -> VH2/1
  [VH4] -> VH4/1
  [VH1] -> VH1/1
  [VH3] -> VH3/1

== system cv_model_F50/RA Cap. ==
  note: 3/2*Tsla > t
  note: Tsla < t < 3/2*Tsla
  note: 0 < t < Tsla
  Constant : Constant
  Constant1 : Constant  Value=pi
  Constant2 : Constant
  Constant3 : Constant  Value=2*pi
  Gain : Gain  Gain=0.5
  Gain1 : Gain  Gain=1.5
  Gain2 : Gain  Gain=0.5
  Math Function{,1..7} (8 alike) : Math  Operator=reciprocal  SignedPower=on
  Sum{1..3,5..6,9} (6 alike) : Sum  Inputs=+-  InputSameDT=on  SaturateOnIntegerOverflow=on  OutDataTypeStr=Inherit: Same as first input
  Sum4 : Sum  InputSameDT=on  SaturateOnIntegerOverflow=on  OutDataTypeStr=Inherit: Same as first input
  Sum7 : Sum  InputSameDT=on  SaturateOnIntegerOverflow=on  OutDataTypeStr=Inherit: Same as first input
  Sum8 : Sum  InputSameDT=on  SaturateOnIntegerOverflow=on  OutDataTypeStr=Inherit: Same as first input
  Switch1 : Switch
  Switch2 : Switch
  Trigonometric Function : Trigonometry  Operator=cos
  Trigonometric Function1 : Trigonometry  Operator=cos
  mult : Product  Inputs=**
  mult1 : Product  Inputs=**/
  mult3 : Product  Inputs=**
  mult4 : Product  Inputs=**/
  Cra : Outport
  tag scope: Cra=global
  wires:
  [Tsla] -> Sum9/2
  Sum9/1 -> Switch1/2
  [Cras_n] -> Math Function/1
  Sum3/1 -> Gain/1
  Gain/1 -> mult/1
  Constant/1 -> Sum1/1
  Trigonometric Function/1 -> Sum1/2
  Constant1/1 -> mult1/1
  mult1/1 -> Trigonometric Function/1
  [Tsla] -> mult1/3
  Sum1/1 -> mult/2
  [t] -> mult1/2
  mult/1 -> Sum7/1
  Math Function/1 -> Sum3/1
  [Crad_n] -> Math Function1/1
  Math Function1/1 -> Sum3/2
  [Crad_n] -> Math Function2/1
  Math Function2/1 -> Sum7/2
  Sum7/1 -> Switch1/3
  [t] -> Sum2/1
  [Tsla] -> Gain1/1
  Gain1/1 -> Sum2/2
  Switch2/1 -> Switch1/1
  Sum2/1 -> Switch2/2
  Sum6/1 -> Gain2/1
  Gain2/1 -> mult3/1
  Constant2/1 -> Sum4/1
  Trigonometric Function1/1 -> Sum4/2
  Constant3/1 -> mult4/1
  mult4/1 -> Trigonometric Function1/1
  [Tsla] -> mult4/3
  Sum4/1 -> mult3/2
  Sum5/1 -> mult4/2
  mult3/1 -> Sum8/1
  [Tsla] -> Sum5/2
  [Cras_n] -> Math Function3/1
  Math Function3/1 -> Sum6/1
  [Crad_n] -> Math Function4/1
  Math Function4/1 -> Sum6/2
  [Crad_n] -> Math Function5/1
  Math Function5/1 -> Sum8/2
  [t] -> Sum5/1
  [t] -> Sum9/1
  Sum8/1 -> Switch2/3
  [Crad_n] -> Math Function6/1
  Math Function6/1 -> Switch2/1
  Switch1/1 -> Math Function7/1
  Math Function7/1 -> [Cra], Cra/1

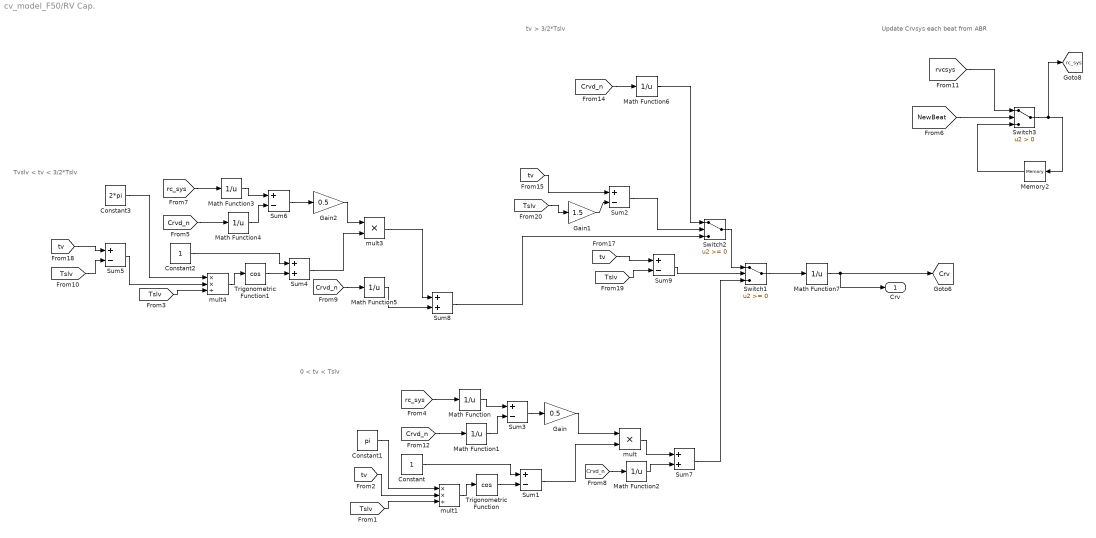
== system cv_model_F50/RV Cap. ==
  note: Update Crvsys each beat from ABR
  note: tv > 3/2*Tslv
  note: Tvslv < tv < 3/2*Tslv
  note: 0 < tv < Tslv
  Constant : Constant
  Constant1 : Constant  Value=pi
  Constant2 : Constant
  Constant3 : Constant  Value=2*pi
  Gain : Gain  Gain=0.5
  Gain1 : Gain  Gain=1.5
  Gain2 : Gain  Gain=0.5
  Math Function{,1..7} (8 alike) : Math  Operator=reciprocal  SignedPower=on
  Memory2 : Memory  InitialCondition=1.2  InheritSampleTime=on
  Sum{1..3,5..6,9} (6 alike) : Sum  Inputs=+-  InputSameDT=on  SaturateOnIntegerOverflow=on  OutDataTypeStr=Inherit: Same as first input
  Sum4 : Sum  InputSameDT=on  SaturateOnIntegerOverflow=on  OutDataTypeStr=Inherit: Same as first input
  Sum7 : Sum  InputSameDT=on  SaturateOnIntegerOverflow=on  OutDataTypeStr=Inherit: Same as first input
  Sum8 : Sum  InputSameDT=on  SaturateOnIntegerOverflow=on  OutDataTypeStr=Inherit: Same as first input
  Switch1 : Switch
  Switch2 : Switch
  Switch3 : Switch  Criteria=u2 > Threshold
  Trigonometric Function : Trigonometry  Operator=cos
  Trigonometric Function1 : Trigonometry  Operator=cos
  mult : Product  Inputs=**
  mult1 : Product  Inputs=**/
  mult3 : Product  Inputs=**
  mult4 : Product  Inputs=**/
  Crv : Outport
  tag scope: Crv=global, rc_sys=global
  wires:
  [Tslv] -> Sum9/2
  Sum9/1 -> Switch1/2
  [rc_sys] -> Math Function/1
  Sum3/1 -> Gain/1
  Gain/1 -> mult/1
  Constant/1 -> Sum1/1
  Trigonometric Function/1 -> Sum1/2
  Constant1/1 -> mult1/1
  mult1/1 -> Trigonometric Function/1
  [Tslv] -> mult1/3
  Sum1/1 -> mult/2
  [tv] -> mult1/2
  mult/1 -> Sum7/1
  Math Function/1 -> Sum3/1
  [Crvd_n] -> Math Function1/1
  Math Function1/1 -> Sum3/2
  [Crvd_n] -> Math Function2/1
  Math Function2/1 -> Sum7/2
  Sum7/1 -> Switch1/3
  [tv] -> Sum2/1
  [Tslv] -> Gain1/1
  Gain1/1 -> Sum2/2
  Switch2/1 -> Switch1/1
  Sum2/1 -> Switch2/2
  Sum6/1 -> Gain2/1
  Gain2/1 -> mult3/1
  Constant2/1 -> Sum4/1
  Trigonometric Function1/1 -> Sum4/2
  Constant3/1 -> mult4/1
  mult4/1 -> Trigonometric Function1/1
  [Tslv] -> mult4/3
  Sum4/1 -> mult3/2
  Sum5/1 -> mult4/2
  mult3/1 -> Sum8/1
  [Tslv] -> Sum5/2
  [rc_sys] -> Math Function3/1
  Math Function3/1 -> Sum6/1
  [Crvd_n] -> Math Function4/1
  Math Function4/1 -> Sum6/2
  [Crvd_n] -> Math Function5/1
  Math Function5/1 -> Sum8/2
  [tv] -> Sum5/1
  [tv] -> Sum9/1
  Sum8/1 -> Switch2/3
  [Crvd_n] -> Math Function6/1
  Math Function6/1 -> Switch2/1
  Switch1/1 -> Math Function7/1
  Math Function7/1 -> [Crv], Crv/1
  [NewBeat] -> Switch3/2
  [rvcsys] -> Switch3/1
  Switch3/1 -> Memory2/1, [rc_sys]
  Memory2/1 -> Switch3/3
